simulink subsystem "ODE_Model"  (R2022b)
settings: Solver=VariableStepAuto  StartTime=0.0  StopTime=10.0  RelTol=1e-3
model mask{pwr=0, Ra=0, La=0, Kphi=0, Be=0, Je=1e-8, Kg=0, enable_Tc=off, tau_c=0, enable_Tsb=off, tau_sb=0, w_sb=0, approximate=off, lambda=1}
  mask prompts: pwr "Vcc - Power Supply [V]:"; Ra "Ra - Armature Resitance [Ohm]:"; La "La - Armature Inductance [H]:"; Kphi "Kphi - Flux Constant [V*s]:"; Be "Be - Viscous Friction [N*m*s]:"; Je "Je - Inertia [Kg*m^2]:"; Kg "Kg - Gear ratio [#]:"; enable_Tc "Coulomb Friction"; tau_c "Tc - Static Friction [N*m]:"; enable_Tsb "Stribeck Friction"; tau_sb "Tsb - Breakaway Torque [N*m]:"; w_sb "w_sb - Breakaway Speed [rad/s]:"; approximate "Approximate sgn with tanh"; lambda "Sigmoid Exponent"
undefined symbols (not defined in the file): motor
settings Model: Creator=gotta  LastModifiedBy=gotta

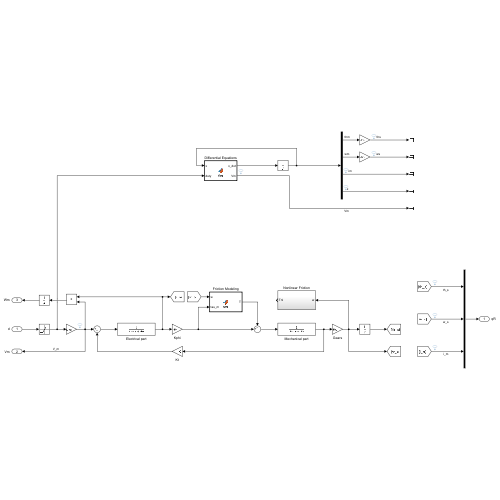
[thumbnail: Simulink's stored preview of the top-level diagram]
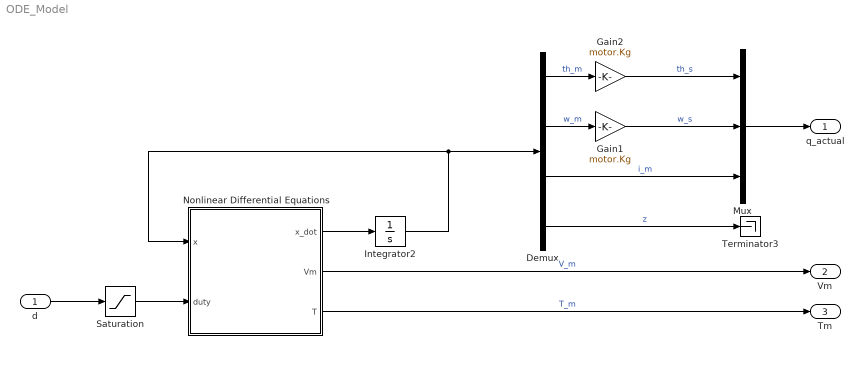
== system ODE_Model ==
  d : Inport
  Demux : Demux
  Gain1 : Gain  Gain=motor.Kg
  Gain2 : Gain  Gain=motor.Kg
  Integrator2 : Integrator  InitialCondition=zeros(4, 1)
  Mux : Mux  Inputs=3
  Nonlinear Differential Equations : MATLAB Function  TreatAsAtomicUnit=on
  Saturation : Saturate  UpperLimit=1  LowerLimit=-1
  Terminator3 : Terminator
  q_actual : Outport
  Vm : Outport  Port=2
  Tm : Outport  Port=3
  wires:
  Mux/1 -> q_actual/1
  d/1 -> Saturation/1
  Saturation/1 -> Nonlinear Differential Equations/2(duty)
  Nonlinear Differential Equations/1(x_dot) -> Integrator2/1
  Integrator2/1 -> Nonlinear Differential Equations/1(x), Demux/1
  Demux/3 -> Mux/3  "i_m"
  Demux/1 -> Gain2/1  "th_m"
  Demux/2 -> Gain1/1  "w_m"
  Demux/4 -> Terminator3/1  "z"
  Gain1/1 -> Mux/2  "w_s"
  Gain2/1 -> Mux/1  "th_s"
  Nonlinear Differential Equations/2(Vm) -> Vm/1  "V_m"
  Nonlinear Differential Equations/3(T) -> Tm/1  "T_m"

== matlab function ODE_Model/Nonlinear Differential Equations ==
  data: x input; duty input; x_dot output; motor parameter; Vm output; T output
function [x_dot, Vm, T] = fcn(x, duty, motor)


thm = x(1);
wm = x(2);
im = x(3);
z = x(4);

xi = 0.1;
sigma_0 = 1;
sigma_1 = 2*xi*sqrt(sigma_0 * motor.Je);

f22 = -(motor.Be + sigma_1) / motor.Je;
f23 = motor.Kphi / motor.Je;
f24 = -sigma_0 / motor.Je;

f32 = -motor.Kphi / motor.La;
f33 = -motor.Ra / motor.La;

F = [
    0, 1,   0,   0;
    0, f22, f23, f24;
    0, f32, f33, 0;
    0, 1,   0,   0; 
    ];

G = [0; 0; motor.Vcc/motor.La; 0];

Ff = motor.tau_c + (motor.tau_sb - motor.tau_c)*exp(-(wm / motor.w_sb)^2);

W = [0; (sigma_1*sigma_0*abs(wm)*z) / (motor.Je*Ff); 0; -(sigma_0*abs(wm)*z) / Ff];



x_dot = F*x + G*duty + W;
Vm = motor.Vcc*duty;
T = sigma_0*z + sigma_1*(wm - sigma_0*abs(wm)*z/Ff) + motor.Be*wm;
